simulink model "ex2"  (R2022b)
settings: Solver=VariableStepAuto  StartTime=0.0  StopTime=stop_time  RelTol=1e-3
undefined symbols (not defined in the file or in its folder): da, dy, r
libraries: cstblocks x2
settings Model: Creator=S280711  LastModifiedBy=franc
settings ModelReferenceCC: EnableRefExpFcnMdlSchedulingChecks=on

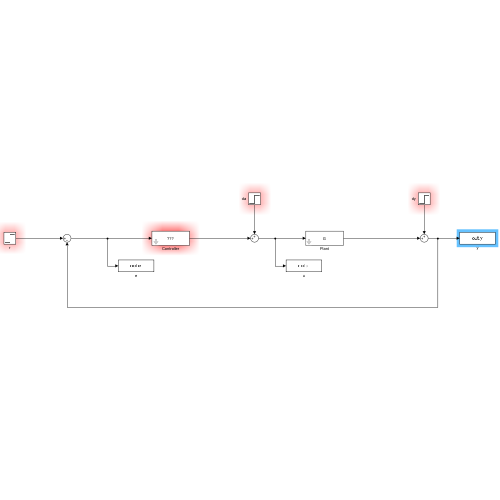
[thumbnail: Simulink's stored preview of the top-level diagram]
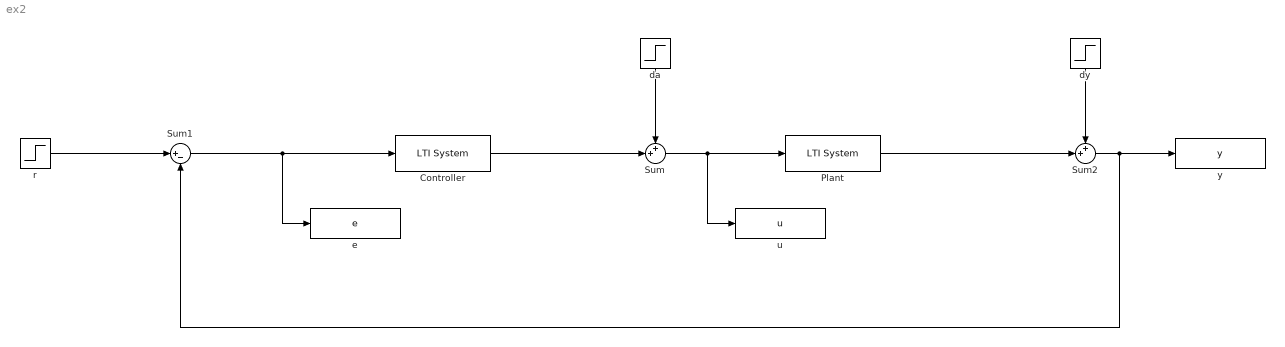
== system ex2 ==
  Controller : cstblocks/LTI System  sys=C  IC=[]
  Plant : cstblocks/LTI System  sys=G  IC=[]
  Sum : Sum  Inputs=++|
  Sum1 : Sum  Inputs=|+-
  Sum2 : Sum  Inputs=++|
  da : Step  Time=0  After=da  SampleTime=0
  dy : Step  Time=0  After=dy  SampleTime=0
  e : ToWorkspace  VariableName=e  SaveFormat=Timeseries  SampleTime=-1
  r : Step  Time=0  After=r  SampleTime=0
  u : ToWorkspace  VariableName=u  SaveFormat=Timeseries  SampleTime=-1
  y : ToWorkspace  VariableName=y  SaveFormat=Timeseries  SampleTime=-1
  wires:
  Sum2/1 -> y/1, Sum1/2
  da/1 -> Sum/1
  dy/1 -> Sum2/1
  r/1 -> Sum1/1
  Sum1/1 -> e/1, Controller/1
  Controller/1 -> Sum/2
  Plant/1 -> Sum2/2
  Sum/1 -> u/1, Plant/1
